simulink library "speedgoatlib_evse"  (R2024b)
settings: Solver=VariableStepAuto  StartTime=0.0  StopTime=10.0  RelTol=1e-3
undefined symbols (not defined in the file): sg_ev_charging_read_m, sg_ev_charging_write_m, sg_ev_isolation_read_m, sg_ev_parameter_read_m, sg_ev_parameter_write_m, sg_ev_precharge_read_m, sg_ev_precharge_write_m, sg_ev_status_m, sg_ev_stop_read_m, sg_ev_stop_write_m, sg_ev_welding_read_m, sg_ev_welding_write_m, sg_evse_charging_read_m, sg_evse_charging_write_m, sg_evse_isolation_read_m, sg_evse_isolation_write_m, sg_evse_parameter_read_m, sg_evse_parameter_write_m, sg_evse_precharge_read_m, sg_evse_precharge_write_m, sg_evse_status_m, sg_evse_stop_read_m, sg_evse_stop_write_m, sg_evse_welding_read_m, sg_evse_welding_write_m
libraries: speedgoatlib_mqtt x199, simulink x39, $bdroot x24
(part 2 of 8)

== system speedgoatlib_evse/Blocks by Charge State/EV Isolation Write  ==
  ready : Inport
  errorcode : Inport  Port=2
  ressSoc : Inport  Port=3
  Compare To Constant : simulink/Logic and Bit Operations/Compare To Constant  relop===  const=1  OutDataTypeStr=boolean
  Compare To Constant1 : simulink/Logic and Bit Operations/Compare To Constant  relop===  const=1  OutDataTypeStr=boolean
  Enabled Subsystem : Subsystem  TreatAsAtomicUnit=on
  Isolation Status Subscribe : speedgoatlib_mqtt/Client/MQTT Client Subscribe  ClientId=parClientId  ConnectionId=parConnectionId  Topic='port0/ci/charge/isolation/status'  QoS=0 - at most once  InitValue=zeros(1,24,'uint8')  Extended=off  SampleTime=parSampleTime
      settings: SourceProductName=MQTT
  Logical Operator : Logic  Operator=OR  AllPortsSameDT=off  OutDataTypeStr=boolean
  Parameter Status Subscribe : speedgoatlib_mqtt/Client/MQTT Client Subscribe  ClientId=parClientId  ConnectionId=parConnectionId  Topic='port0/ci/charge/parameter/status'  QoS=0 - at most once  InitValue=zeros(1,24,'uint8')  Extended=off  SampleTime=parSampleTime
      settings: SourceProductName=MQTT
  string compare logic : Subsystem
  string compare logic1 : $bdroot/Blocks by Charge State/EV Parameter Write /string compare logic  SystemSampleTime=-1  VariantActivationTime=update diagram  EmptyChoice=off  PassThrough=off  PassThroughVariantControl=(default)  EmptyChoiceVariantControl=(default)  AllowFlexibleInterface=on  Latency=0  AutoFrameSizeCalculation=off
  wires:
  string compare logic/1(Out1) -> Compare To Constant1/1
  Isolation Status Subscribe/1 -> string compare logic/1(Input)
  Compare To Constant1/1 -> Logical Operator/2  "Isolation State Reached"
  ready/1 -> Enabled Subsystem/1(ready)
  errorcode/1 -> Enabled Subsystem/2(errorcode)
  ressSoc/1 -> Enabled Subsystem/3(resssoc)
  Parameter Status Subscribe/1 -> string compare logic1/1
  Compare To Constant/1 -> Logical Operator/1  "Parameter State Reached"
  string compare logic1/1 -> Compare To Constant/1
  Logical Operator/1 -> Enabled Subsystem/Enable

== system speedgoatlib_evse/Blocks by Charge State/EV Parameter Read  ==
  Compare To Constant : simulink/Logic and Bit Operations/Compare To Constant  relop===  const=1  OutDataTypeStr=boolean
  Enabled Subsystem : Subsystem  TreatAsAtomicUnit=on
  Parameter Status Subscribe : speedgoatlib_mqtt/Client/MQTT Client Subscribe  ClientId=parClientId  ConnectionId=parConnectionId  Topic='port0/ci/charge/parameter/status'  QoS=0 - at most once  InitValue=zeros(1,24,'uint8')  Extended=off  SampleTime=parSampleTime
      settings: SourceProductName=MQTT
  string compare logic : Subsystem
  Output : Outport
  Output1 : Outport  Port=2
  Output3 : Outport  Port=3
  Output4 : Outport  Port=4
  Output5 : Outport  Port=5
  Output2 : Outport  Port=6
  Output6 : Outport  Port=7
  Output7 : Outport  Port=8
  Output8 : Outport  Port=9
  Output9 : Outport  Port=10
  Output10 : Outport  Port=11
  Output11 : Outport  Port=12
  Output12 : Outport  Port=13
  Output13 : Outport  Port=14
  Output14 : Outport  Port=15
  Output15 : Outport  Port=16
  wires:
  Compare To Constant/1 -> Enabled Subsystem/Enable  "Parameter State Reached"
  string compare logic/1(Out1) -> Compare To Constant/1
  Parameter Status Subscribe/1 -> string compare logic/1(Input)
  Enabled Subsystem/1(SAScheduleTupleID) -> Output/1
  Enabled Subsystem/2(SAScheduleStart) -> Output1/1
  Enabled Subsystem/3(SAScheduleDuration) -> Output3/1
  Enabled Subsystem/4(SASchedulePMax) -> Output4/1
  Enabled Subsystem/5(EVSE Max Voltage Limit) -> Output5/1
  Enabled Subsystem/10(EVSE Current Regulation Tolerance) -> Output9/1
  Enabled Subsystem/9(EVSE Min Voltage Limit) -> Output8/1
  Enabled Subsystem/8(EVSE Min Current Limit) -> Output7/1
  Enabled Subsystem/7(EVSE Max Power Limit) -> Output6/1
  Enabled Subsystem/6(EVSE Max Current Limit) -> Output2/1
  Enabled Subsystem/11(EVSE Peak Current Ripple) -> Output10/1
  Enabled Subsystem/12(EVSE Energy to be Delivered) -> Output11/1
  Enabled Subsystem/13(EVSE Notification Max Delay) -> Output12/1
  Enabled Subsystem/14(EVSE Notification) -> Output13/1
  Enabled Subsystem/15(EVSE Isolationstatus) -> Output14/1
  Enabled Subsystem/16(EVSE Statuscode) -> Output15/1

== system speedgoatlib_evse/Blocks by Charge State/EV Parameter Write  ==
  Input : Inport
  Input1 : Inport  Port=2
  Input2 : Inport  Port=3
  Input3 : Inport  Port=4
  Input4 : Inport  Port=5
  Input5 : Inport  Port=6
  Input6 : Inport  Port=7
  Input7 : Inport  Port=8
  Input8 : Inport  Port=9
  Input9 : Inport  Port=10
  Input10 : Inport  Port=11
  Input11 : Inport  Port=12
  Input12 : Inport  Port=13
  Compare To Constant : simulink/Logic and Bit Operations/Compare To Constant  relop===  const=1  OutDataTypeStr=boolean
  Compare To Constant1 : simulink/Logic and Bit Operations/Compare To Constant  relop===  const=1  OutDataTypeStr=boolean
  Enabled Subsystem : Subsystem  TreatAsAtomicUnit=on
  Init Status Subscribe : speedgoatlib_mqtt/Client/MQTT Client Subscribe  ClientId=parClientId  ConnectionId=parConnectionId  Topic='port0/ci/charge/init/status'  QoS=0 - at most once  InitValue=zeros(1,24,'uint8')  Extended=off  SampleTime=parSampleTime
      settings: SourceProductName=MQTT
  Logical Operator : Logic  Operator=OR  AllPortsSameDT=off  OutDataTypeStr=boolean
  Parameter Status Subscribe : speedgoatlib_mqtt/Client/MQTT Client Subscribe  ClientId=parClientId  ConnectionId=parConnectionId  Topic='port0/ci/charge/parameter/status'  QoS=0 - at most once  InitValue=zeros(1,24,'uint8')  Extended=off  SampleTime=parSampleTime
      settings: SourceProductName=MQTT
  string compare logic : Subsystem
  string compare logic1 : $bdroot/Blocks by Charge State/EV Setup /string compare logic  SystemSampleTime=-1  VariantActivationTime=update diagram  EmptyChoice=off  PassThrough=off  PassThroughVariantControl=(default)  EmptyChoiceVariantControl=(default)  AllowFlexibleInterface=on  Latency=0  AutoFrameSizeCalculation=off
  wires:
  Input12/1 -> Enabled Subsystem/13(bulksoc)
  Input11/1 -> Enabled Subsystem/12(fullsoc)
  Input10/1 -> Enabled Subsystem/11(energyrequest)
  Input5/1 -> Enabled Subsystem/6(maxpowerlimit)
  Input6/1 -> Enabled Subsystem/7(ready)
  Input7/1 -> Enabled Subsystem/8(errorcode)
  Input8/1 -> Enabled Subsystem/9(resssoc)
  Input9/1 -> Enabled Subsystem/10(energycapacity)
  Input4/1 -> Enabled Subsystem/5(mincurrentlimit)
  Input3/1 -> Enabled Subsystem/4(maxcurrentlimit)
  Input2/1 -> Enabled Subsystem/3(maxvoltagelimit)
  Input1/1 -> Enabled Subsystem/2(departuretime)
  Input/1 -> Enabled Subsystem/1(requestedenergytype)
  Parameter Status Subscribe/1 -> string compare logic/1(Input)
  string compare logic/1(Out1) -> Compare To Constant/1
  Compare To Constant/1 -> Logical Operator/2  "Parameter State Reached"
  Compare To Constant1/1 -> Logical Operator/1  "Init State Reached"
  Init Status Subscribe/1 -> string compare logic1/1
  string compare logic1/1 -> Compare To Constant1/1
  Logical Operator/1 -> Enabled Subsystem/Enable

== system speedgoatlib_evse/Blocks by Charge State/EV Pre-Charge Read  ==
  Compare To Constant : simulink/Logic and Bit Operations/Compare To Constant  relop===  const=1  OutDataTypeStr=boolean
  Enabled Subsystem : Subsystem  TreatAsAtomicUnit=on
  Precharge Status Subscribe : speedgoatlib_mqtt/Client/MQTT Client Subscribe  ClientId=parClientId  ConnectionId=parConnectionId  Topic='port0/ci/charge/precharge/status'  QoS=0 - at most once  InitValue=zeros(1,24,'uint8')  Extended=off  SampleTime=parSampleTime
      settings: SourceProductName=MQTT
  string compare logic1 : Subsystem
  evseIsolationstatus : Outport
  evseStatuscode : Outport  Port=2
  evsePresentVoltage : Outport  Port=3
  wires:
  Precharge Status Subscribe/1 -> string compare logic1/1(Input)
  string compare logic1/1(Out1) -> Compare To Constant/1
  Compare To Constant/1 -> Enabled Subsystem/Enable  "Precharge State Reached"
  Enabled Subsystem/1(EVSE Isolationstatus) -> evseIsolationstatus/1
  Enabled Subsystem/2(EVSE Statuscode) -> evseStatuscode/1
  Enabled Subsystem/3(EVSE Present Voltage) -> evsePresentVoltage/1

== system speedgoatlib_evse/Blocks by Charge State/EV Pre-Charge Write  ==
  ready : Inport
  errorcode : Inport  Port=2
  ressSoc : Inport  Port=3
  targetVoltage : Inport  Port=4
  targetCurrent : Inport  Port=5
  Compare To Constant1 : simulink/Logic and Bit Operations/Compare To Constant  relop===  const=1  OutDataTypeStr=boolean
  Compare To Constant2 : simulink/Logic and Bit Operations/Compare To Constant  relop===  const=1  OutDataTypeStr=boolean
  Enabled Subsystem : Subsystem  TreatAsAtomicUnit=on
  Isolation Status Subscribe : speedgoatlib_mqtt/Client/MQTT Client Subscribe  ClientId=parClientId  ConnectionId=parConnectionId  Topic='port0/ci/charge/isolation/status'  QoS=0 - at most once  InitValue=zeros(1,24,'uint8')  Extended=off  SampleTime=parSampleTime
      settings: SourceProductName=MQTT
  Logical Operator : Logic  Operator=OR  AllPortsSameDT=off  OutDataTypeStr=boolean
  Precharge Status Subscribe : speedgoatlib_mqtt/Client/MQTT Client Subscribe  ClientId=parClientId  ConnectionId=parConnectionId  Topic='port0/ci/charge/precharge/status'  QoS=0 - at most once  InitValue=zeros(1,24,'uint8')  Extended=off  SampleTime=parSampleTime
      settings: SourceProductName=MQTT
  string compare logic : Subsystem
  string compare logic1 : $bdroot/Blocks by Charge State/EV Isolation Write /string compare logic  SystemSampleTime=-1  VariantActivationTime=update diagram  EmptyChoice=off  PassThrough=off  PassThroughVariantControl=(default)  EmptyChoiceVariantControl=(default)  AllowFlexibleInterface=on  Latency=0  AutoFrameSizeCalculation=off
  wires:
  targetCurrent/1 -> Enabled Subsystem/5(targetcurrent)
  targetVoltage/1 -> Enabled Subsystem/4(targetvoltage)
  ressSoc/1 -> Enabled Subsystem/3(resssoc)
  errorcode/1 -> Enabled Subsystem/2(errorcode)
  ready/1 -> Enabled Subsystem/1(ready)
  Compare To Constant1/1 -> Logical Operator/2  "Precharge State Reached"
  Precharge Status Subscribe/1 -> string compare logic/1(Input)
  string compare logic/1(Out1) -> Compare To Constant1/1
  string compare logic1/1 -> Compare To Constant2/1
  Isolation Status Subscribe/1 -> string compare logic1/1
  Compare To Constant2/1 -> Logical Operator/1  "Isolation State Reached"
  Logical Operator/1 -> Enabled Subsystem/Enable

== system speedgoatlib_evse/Blocks by Charge State/EV Setup  ==
  Compare To Constant : simulink/Logic and Bit Operations/Compare To Constant  relop===  const=1  OutDataTypeStr=boolean
  Enabled Subsystem : Subsystem  TreatAsAtomicUnit=on
  Init Status Subscribe : speedgoatlib_mqtt/Client/MQTT Client Subscribe  ClientId=parClientId  ConnectionId=parConnectionId  Topic='port0/ci/charge/init/status'  QoS=0 - at most once  InitValue=zeros(1,24,'uint8')  Extended=on  SampleTime=parSampleTime
      settings: SourceProductName=MQTT
  MQTT Client Connection : speedgoatlib_mqtt/Client/MQTT Client Connection  StationId=parClientId  ConnectionId=parConnectionId  IpAddrStr=parRemoteIpAddrStr  TcpPort=parTcpPort  SampleTime=parSampleTime  UserAuthentication=off  Username=''  Password=''
      settings: SourceProductName=MQTT
  MQTT Client Setup : speedgoatlib_mqtt/Client/MQTT Client Setup  StationId=parClientId  ClientIdentifier=parClientIdentifier  IpAddrStr=parIpAddrStr
      settings: SourceProductName=MQTT
  Terminator : Terminator
  Terminator1 : Terminator
  Terminator2 : Terminator
  bulkSoc : Constant  Value=parBulkSoc
  departureTime : Constant  Value=parDepartureTime
  energyCapacity : Constant  Value=parEnergyCapacity
  energyRequest : Constant  Value=parEnergyRequest
  fullSoc : Constant  Value=parFullSoc
  maxCurrentLimit : Constant  Value=parMaxCurrentLimit
  maxPowerLimit : Constant  Value=parMaxPowerLimit
  maxVoltageLimit : Constant  Value=parMaxVoltageLimit
  minCurrentLimit : Constant  Value=parMinCurrentLimit
  ressSoc : Constant  Value=parRessSoc
  string compare logic : Subsystem
  wires:
  Init Status Subscribe/3 -> Terminator1/1
  Init Status Subscribe/1 -> string compare logic/1(Input)
  Init Status Subscribe/2 -> Terminator/1
  string compare logic/1(Out1) -> Compare To Constant/1
  Compare To Constant/1 -> Enabled Subsystem/Enable  "Init State Reached"
  ressSoc/1 -> Enabled Subsystem/6(ressoc)
  maxVoltageLimit/1 -> Enabled Subsystem/2(maxvoltagelimit)
  maxCurrentLimit/1 -> Enabled Subsystem/3(maxcurrentlimit)
  bulkSoc/1 -> Enabled Subsystem/10(bulksoc)
  minCurrentLimit/1 -> Enabled Subsystem/4(mincurrentlimit)
  maxPowerLimit/1 -> Enabled Subsystem/5(maxpowerlimit)
  fullSoc/1 -> Enabled Subsystem/9(fullsoc)
  energyRequest/1 -> Enabled Subsystem/8(energyrequest)
  energyCapacity/1 -> Enabled Subsystem/7(energycapacity)
  departureTime/1 -> Enabled Subsystem/1(departuretime)
  MQTT Client Connection/1 -> Terminator2/1

== system speedgoatlib_evse/Blocks by Charge State/EV Stop Read  ==
  Compare To Constant : simulink/Logic and Bit Operations/Compare To Constant  relop===  const=1  OutDataTypeStr=boolean
  Enabled Subsystem : Subsystem  TreatAsAtomicUnit=on
  Stop Status Subscribe : speedgoatlib_mqtt/Client/MQTT Client Subscribe  ClientId=parClientId  ConnectionId=parConnectionId  Topic='port0/ci/charge/stop/status'  QoS=0 - at most once  InitValue=zeros(1,24,'uint8')  Extended=off  SampleTime=parSampleTime
      settings: SourceProductName=MQTT
  string compare logic : Subsystem
  evseStopProgress : Outport
  evseProcessing : Outport  Port=2
  wires:
  Stop Status Subscribe/1 -> string compare logic/1(Input)
  string compare logic/1(Out1) -> Compare To Constant/1
  Compare To Constant/1 -> Enabled Subsystem/Enable  "Stop State Reached"
  Enabled Subsystem/1(EVSE Stop Progress) -> evseStopProgress/1
  Enabled Subsystem/2(EVSE Processing) -> evseProcessing/1

== system speedgoatlib_evse/Blocks by Charge State/EV Stop Write  ==
  stopProgress : Inport
  Compare To Constant : simulink/Logic and Bit Operations/Compare To Constant  relop===  const=1  OutDataTypeStr=boolean
  Compare To Constant1 : simulink/Logic and Bit Operations/Compare To Constant  relop===  const=1  OutDataTypeStr=boolean
  Enabled Subsystem : Subsystem  TreatAsAtomicUnit=on
  Logical Operator : Logic  Operator=OR  AllPortsSameDT=off  OutDataTypeStr=boolean
  Stop Status Subscribe : speedgoatlib_mqtt/Client/MQTT Client Subscribe  ClientId=parClientId  ConnectionId=parConnectionId  Topic='port0/ci/charge/stop/status'  QoS=0 - at most once  InitValue=zeros(1,24,'uint8')  Extended=off  SampleTime=parSampleTime
      settings: SourceProductName=MQTT
  Welding Status Subscribe : speedgoatlib_mqtt/Client/MQTT Client Subscribe  ClientId=parClientId  ConnectionId=parConnectionId  Topic='port0/ci/charge/welding/status'  QoS=0 - at most once  InitValue=zeros(1,24,'uint8')  Extended=off  SampleTime=parSampleTime
      settings: SourceProductName=MQTT
  string compare logic : Subsystem
  string compare logic1 : $bdroot/Blocks by Charge State/EV Welding Write /string compare logic  SystemSampleTime=-1  VariantActivationTime=update diagram  EmptyChoice=off  PassThrough=off  PassThroughVariantControl=(default)  EmptyChoiceVariantControl=(default)  AllowFlexibleInterface=on  Latency=0  AutoFrameSizeCalculation=off
  wires:
  stopProgress/1 -> Enabled Subsystem/1(stopProgress)
  Compare To Constant/1 -> Logical Operator/2  "Stop State Reached"
  string compare logic/1(Out1) -> Compare To Constant/1
  Stop Status Subscribe/1 -> string compare logic/1(Input)
  Compare To Constant1/1 -> Logical Operator/1  "Welding State Reached"
  string compare logic1/1 -> Compare To Constant1/1
  Welding Status Subscribe/1 -> string compare logic1/1
  Logical Operator/1 -> Enabled Subsystem/Enable

== system speedgoatlib_evse/Blocks by Charge State/EV Welding Read  ==
  Compare To Constant : simulink/Logic and Bit Operations/Compare To Constant  relop===  const=1  OutDataTypeStr=boolean
  Enabled Subsystem : Subsystem  TreatAsAtomicUnit=on
  Welding Status Subscribe : speedgoatlib_mqtt/Client/MQTT Client Subscribe  ClientId=parClientId  ConnectionId=parConnectionId  Topic='port0/ci/charge/welding/status'  QoS=0 - at most once  InitValue=zeros(1,24,'uint8')  Extended=off  SampleTime=parSampleTime
      settings: SourceProductName=MQTT
  string compare logic1 : Subsystem
  evseNotification : Outport
  evseIsolationStatus : Outport  Port=2
  evseStatuscode : Outport  Port=3
  evsePresentVoltage : Outport  Port=4
  wires:
  Enabled Subsystem/4(EVSE Present Voltage) -> evsePresentVoltage/1
  Enabled Subsystem/3(EVSE Statuscode) -> evseStatuscode/1
  Enabled Subsystem/2(EVSE Isolation Status) -> evseIsolationStatus/1
  Enabled Subsystem/1(EVSE Notification) -> evseNotification/1
  Compare To Constant/1 -> Enabled Subsystem/Enable  "Welding State Reached"
  string compare logic1/1(Out1) -> Compare To Constant/1
  Welding Status Subscribe/1 -> string compare logic1/1(Input)

== system speedgoatlib_evse/Blocks by Charge State/EV Welding Write  ==
  ready : Inport
  ressSoc : Inport  Port=2
  errorcode : Inport  Port=3
  Charge Status Subscribe : speedgoatlib_mqtt/Client/MQTT Client Subscribe  Commented=on  ClientId=parClientId  ConnectionId=parConnectionId  Topic='port0/ci/charge/charge/status'  QoS=0 - at most once  InitValue=zeros(1,24,'uint8')  Extended=off  SampleTime=parSampleTime
      settings: SourceProductName=MQTT
  Compare To Constant : simulink/Logic and Bit Operations/Compare To Constant  relop===  const=1  OutDataTypeStr=boolean
  Compare To Constant1 : simulink/Logic and Bit Operations/Compare To Constant  Commented=on  relop===  const=1  OutDataTypeStr=boolean
  Enabled Subsystem : Subsystem  TreatAsAtomicUnit=on
  Logical Operator : Logic  Operator=OR  AllPortsSameDT=off  OutDataTypeStr=boolean
  Welding Status Subscribe : speedgoatlib_mqtt/Client/MQTT Client Subscribe  ClientId=parClientId  ConnectionId=parConnectionId  Topic='port0/ci/charge/welding/status'  QoS=0 - at most once  InitValue=zeros(1,24,'uint8')  Extended=off  SampleTime=parSampleTime
      settings: SourceProductName=MQTT
  string compare logic : Subsystem
  string compare logic1 : $bdroot/Blocks by Charge State/EV Charging Write /string compare logic1  Commented=on  SystemSampleTime=-1  VariantActivationTime=update diagram  EmptyChoice=off  PassThrough=off  PassThroughVariantControl=(default)  EmptyChoiceVariantControl=(default)  AllowFlexibleInterface=on  Latency=0  AutoFrameSizeCalculation=off
  wires:
  Welding Status Subscribe/1 -> string compare logic/1(Input)
  string compare logic/1(Out1) -> Compare To Constant/1
  Compare To Constant/1 -> Logical Operator/2  "Welding State Reached"
  ready/1 -> Enabled Subsystem/1(ready)
  ressSoc/1 -> Enabled Subsystem/3(resssoc)
  errorcode/1 -> Enabled Subsystem/2(errorcode)
  Charge Status Subscribe/1 -> string compare logic1/1
  string compare logic1/1 -> Compare To Constant1/1
  Compare To Constant1/1 -> Logical Operator/1  "Charge State Reached"
  Logical Operator/1 -> Enabled Subsystem/Enable

== system speedgoatlib_evse/Blocks by Charge State/EVSE Charging Read  ==
  Charge Status Subscribe : speedgoatlib_mqtt/Client/MQTT Client Subscribe  ClientId=parClientId  ConnectionId=parConnectionId  Topic='port0/ci/charge/charge/status'  QoS=0 - at most once  InitValue=zeros(1,24,'uint8')  Extended=off  SampleTime=parSampleTime
      settings: SourceProductName=MQTT
  Compare To Constant : simulink/Logic and Bit Operations/Compare To Constant  relop===  const=1  OutDataTypeStr=boolean
  Enabled Subsystem : Subsystem  TreatAsAtomicUnit=on
  string compare logic : Subsystem
  evReady : Outport
  evErrorCode : Outport  Port=2
  evRessSoc : Outport  Port=3
  evTargetVoltage : Outport  Port=4
  evTargetCurrent : Outport  Port=5
  evMaxVoltageLimit : Outport  Port=6
  evMaxCurrentLimit : Outport  Port=7
  evMaxPowerLimit : Outport  Port=8
  evBulkChargingComplete : Outport  Port=9
  evChargingComplete : Outport  Port=10
  evRemainingTimeToBulkSoc : Outport  Port=11
  evRemainingTimeToFullSoc : Outport  Port=12
  wires:
  Compare To Constant/1 -> Enabled Subsystem/Enable  "Charge State Reached"
  string compare logic/1(Out1) -> Compare To Constant/1
  Charge Status Subscribe/1 -> string compare logic/1(Input)
  Enabled Subsystem/1(EV Ready) -> evReady/1
  Enabled Subsystem/2(EV Errorcode) -> evErrorCode/1
  Enabled Subsystem/4(EV Target Voltage) -> evTargetVoltage/1
  Enabled Subsystem/3(EV RESS SOC) -> evRessSoc/1
  Enabled Subsystem/7(EV Max Current Limit) -> evMaxCurrentLimit/1
  Enabled Subsystem/8(EV Max Power Limit) -> evMaxPowerLimit/1
  Enabled Subsystem/6(EV Max Voltage Limit) -> evMaxVoltageLimit/1
  Enabled Subsystem/5(EV Target Current) -> evTargetCurrent/1
  Enabled Subsystem/9(EV Bulk Charging Complete) -> evBulkChargingComplete/1
  Enabled Subsystem/10(EV Charging Complete) -> evChargingComplete/1
  Enabled Subsystem/12(EV Remaining Time to Full SOC) -> evRemainingTimeToFullSoc/1
  Enabled Subsystem/11(EV Remaining Time to Bulk SOC) -> evRemainingTimeToBulkSoc/1

== system speedgoatlib_evse/Blocks by Charge State/EVSE Charging Write  ==
  notification : Inport
  isolationstatus : Inport  Port=2
  statuscode : Inport  Port=3
  presentVoltage : Inport  Port=4
  presentCurrent : Inport  Port=5
  currentLimitAchieved : Inport  Port=6
  voltageLimitAchieved : Inport  Port=7
  powerLimitAchieved : Inport  Port=8
  maxVoltageLimit : Inport  Port=9
  maxCurrentLimit : Inport  Port=10
  maxPowerLimit : Inport  Port=11
  Charge Status Subscribe : speedgoatlib_mqtt/Client/MQTT Client Subscribe  ClientId=parClientId  ConnectionId=parConnectionId  Topic='port0/ci/charge/charge/status'  QoS=0 - at most once  InitValue=zeros(1,24,'uint8')  Extended=off  SampleTime=parSampleTime
      settings: SourceProductName=MQTT
  Compare To Constant : simulink/Logic and Bit Operations/Compare To Constant  relop===  const=1  OutDataTypeStr=boolean
  Compare To Constant1 : simulink/Logic and Bit Operations/Compare To Constant  relop===  const=1  OutDataTypeStr=boolean
  Enabled Subsystem : Subsystem  TreatAsAtomicUnit=on
  Logical Operator : Logic  Operator=OR  AllPortsSameDT=off  OutDataTypeStr=boolean
  Precharge Status Subscribe : speedgoatlib_mqtt/Client/MQTT Client Subscribe  ClientId=parClientId  ConnectionId=parConnectionId  Topic='port0/ci/charge/precharge/status'  QoS=0 - at most once  InitValue=zeros(1,24,'uint8')  Extended=off  SampleTime=parSampleTime
      settings: SourceProductName=MQTT
  string compare logic : Subsystem
  string compare logic1 : $bdroot/Blocks by Charge State/EVSE Pre-Charge Write /string compare logic  SystemSampleTime=-1  VariantActivationTime=update diagram  EmptyChoice=off  PassThrough=off  PassThroughVariantControl=(default)  EmptyChoiceVariantControl=(default)  AllowFlexibleInterface=on  Latency=0  AutoFrameSizeCalculation=off
  wires:
  Charge Status Subscribe/1 -> string compare logic/1(Input)
  string compare logic/1(Out1) -> Compare To Constant/1
  Compare To Constant/1 -> Logical Operator/2  "Charge State Reached"
  presentVoltage/1 -> Enabled Subsystem/4(presentvoltage)
  presentCurrent/1 -> Enabled Subsystem/5(presentcurrent)
  currentLimitAchieved/1 -> Enabled Subsystem/6(currentlimitachieved)
  voltageLimitAchieved/1 -> Enabled Subsystem/7(voltagelimitachieved)
  powerLimitAchieved/1 -> Enabled Subsystem/8(powerlimitachieved)
  maxVoltageLimit/1 -> Enabled Subsystem/9(maxvoltagelimit)
  maxCurrentLimit/1 -> Enabled Subsystem/10(maxcurrentlimit)
  maxPowerLimit/1 -> Enabled Subsystem/11(maxpowerlimit)
  isolationstatus/1 -> Enabled Subsystem/2(isolationstatus)
  notification/1 -> Enabled Subsystem/1(notification)
  statuscode/1 -> Enabled Subsystem/3(statuscode)
  Precharge Status Subscribe/1 -> string compare logic1/1
  string compare logic1/1 -> Compare To Constant1/1
  Compare To Constant1/1 -> Logical Operator/1  "Precharge State Reached"
  Logical Operator/1 -> Enabled Subsystem/Enable

== system speedgoatlib_evse/Blocks by Charge State/EVSE Isolation Read  ==
  Compare To Constant : simulink/Logic and Bit Operations/Compare To Constant  relop===  const=1  OutDataTypeStr=boolean
  Enabled Subsystem : Subsystem  TreatAsAtomicUnit=on
  Isolation Status Subscribe : speedgoatlib_mqtt/Client/MQTT Client Subscribe  ClientId=parClientId  ConnectionId=parConnectionId  Topic='port0/ci/charge/isolation/status'  QoS=0 - at most once  InitValue=zeros(1,24,'uint8')  Extended=off  SampleTime=parSampleTime
      settings: SourceProductName=MQTT
  string compare logic : Subsystem
  evReady : Outport
  evErrorCode : Outport  Port=2
  evRessSoc : Outport  Port=3
  wires:
  Compare To Constant/1 -> Enabled Subsystem/Enable  "Isolation State Reached"
  string compare logic/1(Out1) -> Compare To Constant/1
  Isolation Status Subscribe/1 -> string compare logic/1(Input)
  Enabled Subsystem/1(EV Ready) -> evReady/1
  Enabled Subsystem/2(EV Errorcode) -> evErrorCode/1
  Enabled Subsystem/3(EV RESS SOC) -> evRessSoc/1

== system speedgoatlib_evse/Blocks by Charge State/EVSE Isolation Write  ==
  evseProcessing : Inport
  isolationStatus : Inport  Port=2
  statusCode : Inport  Port=3
  Compare To Constant : simulink/Logic and Bit Operations/Compare To Constant  relop===  const=1  OutDataTypeStr=boolean
  Compare To Constant1 : simulink/Logic and Bit Operations/Compare To Constant  relop===  const=1  OutDataTypeStr=boolean
  Enabled Subsystem : Subsystem  TreatAsAtomicUnit=on
  Isolation Status Subscribe : speedgoatlib_mqtt/Client/MQTT Client Subscribe  ClientId=parClientId  ConnectionId=parConnectionId  Topic='port0/ci/charge/isolation/status'  QoS=0 - at most once  InitValue=zeros(1,24,'uint8')  Extended=off  SampleTime=parSampleTime
      settings: SourceProductName=MQTT
  Logical Operator : Logic  Operator=OR  AllPortsSameDT=off  OutDataTypeStr=boolean
  Parameter Status Subscribe : speedgoatlib_mqtt/Client/MQTT Client Subscribe  ClientId=parClientId  ConnectionId=parConnectionId  Topic='port0/ci/charge/parameter/status'  QoS=0 - at most once  InitValue=zeros(1,24,'uint8')  Extended=off  SampleTime=parSampleTime
      settings: SourceProductName=MQTT
  string compare logic : Subsystem
  string compare logic1 : $bdroot/Blocks by Charge State/EVSE Parameter Write /string compare logic  SystemSampleTime=-1  VariantActivationTime=update diagram  EmptyChoice=off  PassThrough=off  PassThroughVariantControl=(default)  EmptyChoiceVariantControl=(default)  AllowFlexibleInterface=on  Latency=0  AutoFrameSizeCalculation=off
  wires:
  evseProcessing/1 -> Enabled Subsystem/1(evseprocessing)
  statusCode/1 -> Enabled Subsystem/3(statuscode)
  isolationStatus/1 -> Enabled Subsystem/2(isolationstatus)
  Compare To Constant/1 -> Logical Operator/2  "Isolation State Reached"
  string compare logic/1(Out1) -> Compare To Constant/1
  Isolation Status Subscribe/1 -> string compare logic/1(Input)
  Parameter Status Subscribe/1 -> string compare logic1/1
  string compare logic1/1 -> Compare To Constant1/1
  Compare To Constant1/1 -> Logical Operator/1  "Parameter State Reached"
  Logical Operator/1 -> Enabled Subsystem/Enable

== system speedgoatlib_evse/Blocks by Charge State/EVSE Parameter Read  ==
  Compare To Constant : simulink/Logic and Bit Operations/Compare To Constant  relop===  const=1  OutDataTypeStr=boolean
  Enabled Subsystem : Subsystem  TreatAsAtomicUnit=on
  Parameter Status Subscribe : speedgoatlib_mqtt/Client/MQTT Client Subscribe  ClientId=parClientId  ConnectionId=parConnectionId  Topic='port0/ci/charge/parameter/status'  QoS=0 - at most once  InitValue=zeros(1,24,'uint8')  Extended=off  SampleTime=parSampleTime
      settings: SourceProductName=MQTT
  string compare logic : Subsystem
  Output : Outport
  Output1 : Outport  Port=2
  Output3 : Outport  Port=3
  Output4 : Outport  Port=4
  Output5 : Outport  Port=5
  Output6 : Outport  Port=6
  Output7 : Outport  Port=7
  Output8 : Outport  Port=8
  Output9 : Outport  Port=9
  Output10 : Outport  Port=10
  Output11 : Outport  Port=11
  Output12 : Outport  Port=12
  Output13 : Outport  Port=13
  wires:
  Parameter Status Subscribe/1 -> string compare logic/1(Input)
  string compare logic/1(Out1) -> Compare To Constant/1
  Compare To Constant/1 -> Enabled Subsystem/Enable  "Parameter State Reached"
  Enabled Subsystem/1(EV requestedenergytype) -> Output/1
  Enabled Subsystem/2(EV departuretime) -> Output1/1
  Enabled Subsystem/3(EV Max Voltage Limit) -> Output3/1
  Enabled Subsystem/6(EV Max Power Limit) -> Output6/1
  Enabled Subsystem/7(EV Ready) -> Output7/1
  Enabled Subsystem/5(EV Min Current Limit) -> Output5/1
  Enabled Subsystem/4(EV Max Current Limit) -> Output4/1
  Enabled Subsystem/10(EV energycapacity) -> Output10/1
  Enabled Subsystem/11(EV energyrequest) -> Output11/1
  Enabled Subsystem/13(EV Bulksoc) -> Output13/1
  Enabled Subsystem/12(EV Fullsoc) -> Output12/1
  Enabled Subsystem/8(EV Errorcode) -> Output8/1
  Enabled Subsystem/9(EV RessSoc) -> Output9/1

== system speedgoatlib_evse/Blocks by Charge State/EVSE Parameter Write  ==
  Input : Inport
  Input1 : Inport  Port=2
  Input2 : Inport  Port=3
  Input3 : Inport  Port=4
  Input4 : Inport  Port=5
  Input5 : Inport  Port=6
  Input6 : Inport  Port=7
  Input7 : Inport  Port=8
  Input8 : Inport  Port=9
  Input9 : Inport  Port=10
  Input10 : Inport  Port=11
  Input11 : Inport  Port=12
  Input12 : Inport  Port=13
  Input13 : Inport  Port=14
  Input14 : Inport  Port=15
  Input15 : Inport  Port=16
  Input16 : Inport  Port=17
  Compare To Constant : simulink/Logic and Bit Operations/Compare To Constant  relop===  const=1  OutDataTypeStr=boolean
  Compare To Constant1 : simulink/Logic and Bit Operations/Compare To Constant  relop===  const=1  OutDataTypeStr=boolean
  Enabled Subsystem : Subsystem  TreatAsAtomicUnit=on
  Init Status Subscribe : speedgoatlib_mqtt/Client/MQTT Client Subscribe  ClientId=parClientId  ConnectionId=parConnectionId  Topic='port0/ci/charge/init/status'  QoS=0 - at most once  InitValue=zeros(1,24,'uint8')  Extended=off  SampleTime=parSampleTime
      settings: SourceProductName=MQTT
  Logical Operator : Logic  Operator=OR  AllPortsSameDT=off  OutDataTypeStr=boolean
  Parameter Status Subscribe : speedgoatlib_mqtt/Client/MQTT Client Subscribe  ClientId=parClientId  ConnectionId=parConnectionId  Topic='port0/ci/charge/parameter/status'  QoS=0 - at most once  InitValue=zeros(1,24,'uint8')  Extended=off  SampleTime=parSampleTime
      settings: SourceProductName=MQTT
  string compare logic : Subsystem
  string compare logic1 : $bdroot/Blocks by Charge State/EVSE Setup /string compare logic  SystemSampleTime=-1  VariantActivationTime=update diagram  EmptyChoice=off  PassThrough=off  PassThroughVariantControl=(default)  EmptyChoiceVariantControl=(default)  AllowFlexibleInterface=on  Latency=0  AutoFrameSizeCalculation=off
  wires:
  Input4/1 -> Enabled Subsystem/5(SAschedulePMax)
  Input3/1 -> Enabled Subsystem/4(SAscheduleDuration)
  Input2/1 -> Enabled Subsystem/3(SAscheduleStart)
  Input1/1 -> Enabled Subsystem/2(SAscheduleID)
  Input/1 -> Enabled Subsystem/1(evseprocessing)
  Input14/1 -> Enabled Subsystem/15(notification)
  Input15/1 -> Enabled Subsystem/16(isolationstatus)
  Input16/1 -> Enabled Subsystem/17(statuscode)
  Input13/1 -> Enabled Subsystem/14(notificationmaxdelay)
  Input12/1 -> Enabled Subsystem/13(energytobedelivered)
  Input6/1 -> Enabled Subsystem/7(maxcurrentlimit)
  Input7/1 -> Enabled Subsystem/8(maxpowerlimit)
  Input8/1 -> Enabled Subsystem/9(minvoltagelimit)
  Input11/1 -> Enabled Subsystem/12(peakcurrentripple)
  Input10/1 -> Enabled Subsystem/11(currentregtolerance)
  Input9/1 -> Enabled Subsystem/10(mincurrentlimit)
  Input5/1 -> Enabled Subsystem/6(maxvoltagelimit)
  Compare To Constant/1 -> Logical Operator/2  "Parameter State Reached"
  string compare logic/1(Out1) -> Compare To Constant/1
  Parameter Status Subscribe/1 -> string compare logic/1(Input)
  string compare logic1/1 -> Compare To Constant1/1
  Compare To Constant1/1 -> Logical Operator/1  "Init State Reached"
  Init Status Subscribe/1 -> string compare logic1/1
  Logical Operator/1 -> Enabled Subsystem/Enable

== system speedgoatlib_evse/Blocks by Charge State/EVSE Pre-Charge Read  ==
  Compare To Constant : simulink/Logic and Bit Operations/Compare To Constant  relop===  const=1  OutDataTypeStr=boolean
  Enabled Subsystem : Subsystem  TreatAsAtomicUnit=on
  Precharge Status Subscribe : speedgoatlib_mqtt/Client/MQTT Client Subscribe  ClientId=parClientId  ConnectionId=parConnectionId  Topic='port0/ci/charge/precharge/status'  QoS=0 - at most once  InitValue=zeros(1,24,'uint8')  Extended=off  SampleTime=parSampleTime
      settings: SourceProductName=MQTT
  string compare logic : Subsystem
  evReady : Outport
  evErrorCode : Outport  Port=2
  evRessSoc : Outport  Port=3
  evTargetVoltage : Outport  Port=4
  evTargetCurrent : Outport  Port=5
  wires:
  Compare To Constant/1 -> Enabled Subsystem/Enable  "Precharge State Reached"
  string compare logic/1(Out1) -> Compare To Constant/1
  Precharge Status Subscribe/1 -> string compare logic/1(Input)
  Enabled Subsystem/1(EV Ready) -> evReady/1
  Enabled Subsystem/2(EV Errorcode) -> evErrorCode/1
  Enabled Subsystem/4(EV Target Voltage) -> evTargetVoltage/1
  Enabled Subsystem/3(EV RESS SOC) -> evRessSoc/1
  Enabled Subsystem/5(EV Target Current) -> evTargetCurrent/1

== system speedgoatlib_evse/Blocks by Charge State/EVSE Pre-Charge Write  ==
  isolationStatus : Inport
  statusCode : Inport  Port=2
  presentVoltage : Inport  Port=3
  Compare To Constant : simulink/Logic and Bit Operations/Compare To Constant  relop===  const=1  OutDataTypeStr=boolean
  Compare To Constant1 : simulink/Logic and Bit Operations/Compare To Constant  relop===  const=1  OutDataTypeStr=boolean
  Enabled Subsystem : Subsystem  TreatAsAtomicUnit=on
  Isolation Status Subscribe : speedgoatlib_mqtt/Client/MQTT Client Subscribe  ClientId=parClientId  ConnectionId=parConnectionId  Topic='port0/ci/charge/isolation/status'  QoS=0 - at most once  InitValue=zeros(1,24,'uint8')  Extended=off  SampleTime=parSampleTime
      settings: SourceProductName=MQTT
  Logical Operator : Logic  Operator=OR  AllPortsSameDT=off  OutDataTypeStr=boolean
  Precharge Status Subscribe : speedgoatlib_mqtt/Client/MQTT Client Subscribe  ClientId=parClientId  ConnectionId=parConnectionId  Topic='port0/ci/charge/precharge/status'  QoS=0 - at most once  InitValue=zeros(1,24,'uint8')  Extended=off  SampleTime=parSampleTime
      settings: SourceProductName=MQTT
  string compare logic : Subsystem
  string compare logic1 : $bdroot/Blocks by Charge State/EVSE Isolation Write /string compare logic  SystemSampleTime=-1  VariantActivationTime=update diagram  EmptyChoice=off  PassThrough=off  PassThroughVariantControl=(default)  EmptyChoiceVariantControl=(default)  AllowFlexibleInterface=on  Latency=0  AutoFrameSizeCalculation=off
  wires:
  Precharge Status Subscribe/1 -> string compare logic/1(Input)
  string compare logic/1(Out1) -> Compare To Constant/1
  Compare To Constant/1 -> Logical Operator/2  "Precharge State Reached"
  isolationStatus/1 -> Enabled Subsystem/1(isolationstatus)
  statusCode/1 -> Enabled Subsystem/2(statuscode)
  presentVoltage/1 -> Enabled Subsystem/3(presentvoltage)
  string compare logic1/1 -> Compare To Constant1/1
  Isolation Status Subscribe/1 -> string compare logic1/1
  Compare To Constant1/1 -> Logical Operator/1  "Isolation State Reached"
  Logical Operator/1 -> Enabled Subsystem/Enable

== system speedgoatlib_evse/Blocks by Charge State/EVSE Setup  ==
  Compare To Constant : simulink/Logic and Bit Operations/Compare To Constant  relop===  const=1  OutDataTypeStr=boolean
  Enabled Subsystem : Subsystem  TreatAsAtomicUnit=on
  Init Status Subscribe : speedgoatlib_mqtt/Client/MQTT Client Subscribe  ClientId=parClientId  ConnectionId=parConnectionId  Topic='port0/ci/charge/init/status'  QoS=0 - at most once  InitValue=zeros(1,24,'uint8')  Extended=on  SampleTime=parSampleTime
      settings: SourceProductName=MQTT
  MQTT Client Connection : speedgoatlib_mqtt/Client/MQTT Client Connection  StationId=parClientId  ConnectionId=parConnectionId  IpAddrStr=parRemoteIpAddrStr  TcpPort=parTcpPort  SampleTime=parSampleTime  UserAuthentication=off  Username=''  Password=''
      settings: SourceProductName=MQTT
  MQTT Client Setup : speedgoatlib_mqtt/Client/MQTT Client Setup  StationId=parClientId  ClientIdentifier=parClientIdentifier  IpAddrStr=parIpAddrStr
      settings: SourceProductName=MQTT
  Terminator : Terminator
  Terminator1 : Terminator
  Terminator2 : Terminator
  currentRegulationTolerance : Constant  Value=parCurrRegTol
  maxCurrentLimit : Constant  Value=parMaxCurrentLimit
  maxPowerLimit : Constant  Value=parMaxPowerLimit
  maxVoltageLimit : Constant  Value=parMaxVoltageLimit
  minCurrentLimit : Constant  Value=parMinCurrentLimit
  minVoltageLimit : Constant  Value=parMinVoltageLimit
  peakCurrentRipple : Constant  Value=parPeakCurrentRipple
  string compare logic : Subsystem
  wires:
  Init Status Subscribe/3 -> Terminator1/1
  Init Status Subscribe/1 -> string compare logic/1(Input)
  Init Status Subscribe/2 -> Terminator/1
  string compare logic/1(Out1) -> Compare To Constant/1
  Compare To Constant/1 -> Enabled Subsystem/Enable  "Init State Reached"
  maxVoltageLimit/1 -> Enabled Subsystem/1(maxvoltagelimit)
  maxCurrentLimit/1 -> Enabled Subsystem/2(maxcurrentlimit)
  minCurrentLimit/1 -> Enabled Subsystem/3(mincurrentlimit)
  maxPowerLimit/1 -> Enabled Subsystem/4(maxpowerlimit)
  MQTT Client Connection/1 -> Terminator2/1
  minVoltageLimit/1 -> Enabled Subsystem/5(minvoltagelimit)
  currentRegulationTolerance/1 -> Enabled Subsystem/6(currentregtolerance)
  peakCurrentRipple/1 -> Enabled Subsystem/7(peakcurrentripple)

== system speedgoatlib_evse/Blocks by Charge State/EVSE Stop Read  ==
  Compare To Constant : simulink/Logic and Bit Operations/Compare To Constant  relop===  const=1  OutDataTypeStr=boolean
  Enabled Subsystem : Subsystem  TreatAsAtomicUnit=on
  Stop Status Subscribe : speedgoatlib_mqtt/Client/MQTT Client Subscribe  ClientId=parClientId  ConnectionId=parConnectionId  Topic='port0/ci/charge/stop/status'  QoS=0 - at most once  InitValue=zeros(1,24,'uint8')  Extended=off  SampleTime=parSampleTime
      settings: SourceProductName=MQTT
  string compare logic : Subsystem
  evStopProgress : Outport
  wires:
  Compare To Constant/1 -> Enabled Subsystem/Enable  "Stop State Reached"
  string compare logic/1(Out1) -> Compare To Constant/1
  Stop Status Subscribe/1 -> string compare logic/1(Input)
  Enabled Subsystem/1(EV Stop Progress) -> evStopProgress/1

== system speedgoatlib_evse/Blocks by Charge State/EVSE Stop Write  ==
  stopProgress : Inport
  evseProcessing : Inport  Port=2
  Compare To Constant : simulink/Logic and Bit Operations/Compare To Constant  relop===  const=1  OutDataTypeStr=boolean
  Compare To Constant1 : simulink/Logic and Bit Operations/Compare To Constant  relop===  const=1  OutDataTypeStr=boolean
  Enabled Subsystem : Subsystem  TreatAsAtomicUnit=on
  Logical Operator : Logic  Operator=OR  AllPortsSameDT=off  OutDataTypeStr=boolean
  Stop Status Subscribe : speedgoatlib_mqtt/Client/MQTT Client Subscribe  ClientId=parClientId  ConnectionId=parConnectionId  Topic='port0/ci/charge/stop/status'  QoS=0 - at most once  InitValue=zeros(1,24,'uint8')  Extended=off  SampleTime=parSampleTime
      settings: SourceProductName=MQTT
  Welding Status Subscribe : speedgoatlib_mqtt/Client/MQTT Client Subscribe  ClientId=parClientId  ConnectionId=parConnectionId  Topic='port0/ci/charge/welding/status'  QoS=0 - at most once  InitValue=zeros(1,24,'uint8')  Extended=off  SampleTime=parSampleTime
      settings: SourceProductName=MQTT
  string compare logic : Subsystem
  string compare logic1 : $bdroot/Blocks by Charge State/EVSE Welding Write /string compare logic  SystemSampleTime=-1  VariantActivationTime=update diagram  EmptyChoice=off  PassThrough=off  PassThroughVariantControl=(default)  EmptyChoiceVariantControl=(default)  AllowFlexibleInterface=on  Latency=0  AutoFrameSizeCalculation=off
  wires:
  Stop Status Subscribe/1 -> string compare logic/1(Input)
  string compare logic/1(Out1) -> Compare To Constant/1
  Compare To Constant/1 -> Logical Operator/2  "Stop State Reached"
  stopProgress/1 -> Enabled Subsystem/1(stopProgress)
  evseProcessing/1 -> Enabled Subsystem/2(evseProcessing)
  string compare logic1/1 -> Compare To Constant1/1
  Compare To Constant1/1 -> Logical Operator/1  "Welding State Reached"
  Welding Status Subscribe/1 -> string compare logic1/1
  Logical Operator/1 -> Enabled Subsystem/Enable

== system speedgoatlib_evse/Blocks by Charge State/EVSE Welding Read  ==
  Compare To Constant : simulink/Logic and Bit Operations/Compare To Constant  relop===  const=1  OutDataTypeStr=boolean
  Enabled Subsystem : Subsystem  TreatAsAtomicUnit=on
  Welding Status Subscribe : speedgoatlib_mqtt/Client/MQTT Client Subscribe  ClientId=parClientId  ConnectionId=parConnectionId  Topic='port0/ci/charge/welding/status'  QoS=0 - at most once  InitValue=zeros(1,24,'uint8')  Extended=off  SampleTime=parSampleTime
      settings: SourceProductName=MQTT
  string compare logic : Subsystem
  evReady : Outport
  evErrorCode : Outport  Port=2
  evRessSoc : Outport  Port=3
  wires:
  Enabled Subsystem/3(EV RESS SOC) -> evRessSoc/1
  Enabled Subsystem/2(EV Errorcode) -> evErrorCode/1
  Enabled Subsystem/1(EV Ready) -> evReady/1
  Welding Status Subscribe/1 -> string compare logic/1(Input)
  string compare logic/1(Out1) -> Compare To Constant/1
  Compare To Constant/1 -> Enabled Subsystem/Enable  "Welding State Reached"

== system speedgoatlib_evse/Blocks by Charge State/EVSE Welding Write  ==
  notification : Inport
  isolationstatus : Inport  Port=2
  statuscode : Inport  Port=3
  presentVoltage : Inport  Port=4
  Charge Status Subscribe : speedgoatlib_mqtt/Client/MQTT Client Subscribe  Commented=on  ClientId=parClientId  ConnectionId=parConnectionId  Topic='port0/ci/charge/charge/status'  QoS=0 - at most once  InitValue=zeros(1,24,'uint8')  Extended=off  SampleTime=parSampleTime
      settings: SourceProductName=MQTT
  Compare To Constant : simulink/Logic and Bit Operations/Compare To Constant  relop===  const=1  OutDataTypeStr=boolean
  Compare To Constant1 : simulink/Logic and Bit Operations/Compare To Constant  Commented=on  relop===  const=1  OutDataTypeStr=boolean
  Enabled Subsystem : Subsystem  TreatAsAtomicUnit=on
  Logical Operator : Logic  Operator=OR  AllPortsSameDT=off  OutDataTypeStr=boolean
  Welding Status Subscribe : speedgoatlib_mqtt/Client/MQTT Client Subscribe  ClientId=parClientId  ConnectionId=parConnectionId  Topic='port0/ci/charge/welding/status'  QoS=0 - at most once  InitValue=zeros(1,24,'uint8')  Extended=off  SampleTime=parSampleTime
      settings: SourceProductName=MQTT
  string compare logic : Subsystem
  string compare logic1 : $bdroot/Blocks by Charge State/EVSE Charging Write /string compare logic  Commented=on  SystemSampleTime=-1  VariantActivationTime=update diagram  EmptyChoice=off  PassThrough=off  PassThroughVariantControl=(default)  EmptyChoiceVariantControl=(default)  AllowFlexibleInterface=on  Latency=0  AutoFrameSizeCalculation=off
  wires:
  statuscode/1 -> Enabled Subsystem/3(statuscode)
  isolationstatus/1 -> Enabled Subsystem/2(isolationstatus)
  notification/1 -> Enabled Subsystem/1(notification)
  presentVoltage/1 -> Enabled Subsystem/4(presentvoltage)
  Compare To Constant/1 -> Logical Operator/2  "Welding State Reached"
  string compare logic/1(Out1) -> Compare To Constant/1
  Welding Status Subscribe/1 -> string compare logic/1(Input)
  Charge Status Subscribe/1 -> string compare logic1/1
  string compare logic1/1 -> Compare To Constant1/1
  Compare To Constant1/1 -> Logical Operator/1  "Charge State Reached"
  Logical Operator/1 -> Enabled Subsystem/Enable
